simulink library "inp"  (R2021b)
settings: Solver=VariableStepAuto  StartTime=0.0  StopTime=10.0  RelTol=1e-3
undefined symbols (not defined in the file): C_TASK_5MS_S, FALSE, KINP_AcoreReadyToSlp_flg_ovrdflg, KINP_AcoreReadyToSlp_flg_ovrdval, KINP_AllowMovThd_OTA_enum_ovrdflg, KINP_AllowMovThd_OTA_enum_ovrdval, KINP_APSAngleTarget_Deg_ovrdflg, KINP_APSAngleTarget_Deg_ovrdval, KINP_APSDecReq_mps2_ovrdflg, KINP_APSDecReq_mps2_ovrdval, KINP_APSDecReqA_flg_ovrdflg, KINP_APSDecReqA_flg_ovrdval, KINP_APSDFLL_cm_ovrdflg, KINP_APSDFLL_cm_ovrdval, KINP_APSDFLR_cm_ovrdflg, KINP_APSDFLR_cm_ovrdval, KINP_APSDRLL_cm_ovrdflg, KINP_APSDRLL_cm_ovrdval, KINP_APSDRLR_cm_ovrdflg, KINP_APSDRLR_cm_ovrdval, KINP_APSExitCondition_enum_ovrdflg, KINP_APSExitCondition_enum_ovrdval, KINP_APSHWVer_enum_ovrdflg, KINP_APSHWVer_enum_ovrdval, KINP_APSProgressPCT_pct_ovrdflg, KINP_APSProgressPCT_pct_ovrdval, KINP_APSReq_enum_ovrdflg, KINP_APSReq_enum_ovrdval, KINP_APSRQDisplay_enum_ovrdflg, KINP_APSRQDisplay_enum_ovrdval, KINP_APSRqEPASCtrl_flg_ovrdflg, KINP_APSRqEPASCtrl_flg_ovrdval, KINP_APSShiftPosnReq_enum_ovrdval, KINP_APSShiftPosnReq_enum_ovrflg, KINP_APSSpeedCMD_kph_ovrdval, KINP_APSSpeedCMD_kph_ovrflg, KINP_APSStaSystem_enum_ovrdflg, KINP_APSStaSystem_enum_ovrdval, KINP_APSSWVer_enum_ovrdflg, KINP_APSSWVer_enum_ovrdval, KINP_APSVMCReqA_flg_ovrdval, KINP_APSVMCReqA_flg_ovrflg, KINP_APSVRqEPASCtrl_flg_ovrdflg, KINP_APSVRqEPASCtrl_flg_ovrdval, KINP_AuxBattVolmV_mV_ovrdflg, KINP_AuxBattVolmV_mV_ovrdval, KINP_CAASSta_enum_ovrdflg, KINP_CAASSta_enum_ovrdval, KINP_CAASVMCReqA_flg_ovrdval, KINP_CAASVMCReqA_flg_ovrflg, KINP_Chime_enum_ovrdflg, KINP_Chime_enum_ovrdval, KINP_ClearDTCcmd_flg_ovrdflg, KINP_ClearDTCcmd_flg_ovrdval, KINP_EvccAplusPwrUpReq_flg_ovrdflg, KINP_EvccAplusPwrUpReq_flg_ovrdval, KINP_LFID_raw_ovrdval, KINP_LFID_raw_ovrflg, KINP_LRID_raw_ovrdval, KINP_MemOffsetAccX_raw16_ovrdflg ... (+118)
libraries: FVT_lib x595, hcu_lib x1
(part 4 of 27)

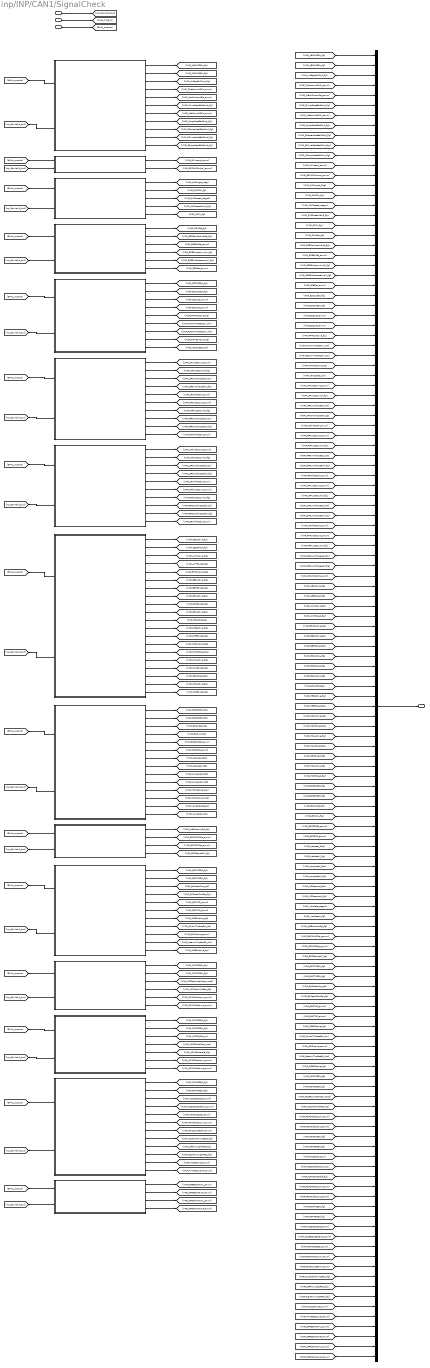
== system inp/INP/CAN1/SignalCheck ==
  inp_CanValid_bus : Inport
  TASK_TIME_S : Inport  Port=2
  BHAL_outputs : Inport  Port=3
  ABM1 : Subsystem
  EPAS1 : Subsystem
  EPAS2 : Subsystem
  EPB1 : Subsystem
  ESC1 : Subsystem
  ESC2 : Subsystem
  ESC3 : Subsystem
  ESC4 : Subsystem
  ESC5 : Subsystem
  ESC6 : Subsystem
  ESC7 : Subsystem
  FCM2 : Subsystem
  FCM3 : Subsystem
  FCM4 : Subsystem
  SRR1 : Subsystem
  bus_creator : BusCreator  Inputs=131
  inp_Hal_bus : Outport
  wires:
  inp_CanValid_bus/1 -> [inp_CanValid_bus]
  TASK_TIME_S/1 -> [TASK_TIME_S]
  BHAL_outputs/1 -> [BHAL_outputs]
  [BHAL_outputs] -> ABM1/1(BHAL_outputs)
  [inp_CanValid_bus] -> ABM1/2(inp_CanValid_bus)
  ABM1/1(VINP_ABM1CSErr_flg) -> [VINP_ABM1CSErr_flg]
  ABM1/2(VINP_ABM1RCErr_flg) -> [VINP_ABM1RCErr_flg]
  ABM1/3(VINP_AirBagFailCmd_flg) -> [VINP_AirBagFailCmd_flg]
  ABM1/4(VINP_ChecksumABM1_enum) -> [VINP_ChecksumABM1_enum]
  ABM1/5(VINP_CrashOutputSts_enum) -> [VINP_CrashOutputSts_enum]
  ABM1/6(VINP_DriverSeatBeltCmd_flg) -> [VINP_DriverSeatBeltCmd_flg]
  ABM1/7(VINP_LifeCountABM1_enum) -> [VINP_LifeCountABM1_enum]
  ABM1/8(VINP_PsngrSeatBeltCmd_flg) -> [VINP_PsngrSeatBeltCmd_flg]
  ABM1/9(VINP_RCenterSeatBeltCmd_flg) -> [VINP_RCenterSeatBeltCmd_flg]
  ABM1/10(VINP_RDriverSeatBeltCmd_flg) -> [VINP_RDriverSeatBeltCmd_flg]
  ABM1/11(VINP_RPsngrSeatBeltCmd_flg) -> [VINP_RPsngrSeatBeltCmd_flg]
  [BHAL_outputs] -> EPAS1/1(BHAL_outputs)
  [inp_CanValid_bus] -> EPAS1/2(inp_CanValid_bus)
  EPAS1/1(VINP_DriIntend_enum) -> [VINP_DriIntend_enum]
  EPAS1/2(VINP_EPSAOIControl_enum) -> [VINP_EPSAOIControl_enum]
  [BHAL_outputs] -> EPAS2/1(BHAL_outputs)
  [inp_CanValid_bus] -> EPAS2/2(inp_CanValid_bus)
  EPAS2/1(VINP_SASAngle_Deg) -> [VINP_SASAngle_Deg]
  EPAS2/2(VINP_SASCAL_flg) -> [VINP_SASCAL_flg]
  EPAS2/3(VINP_SASSpeed_degps) -> [VINP_SASSpeed_degps]
  EPAS2/4(VINP_SASSpeedValid_flg) -> [VINP_SASSpeedValid_flg]
  EPAS2/5(VINP_SASV_flg) -> [VINP_SASV_flg]
  [BHAL_outputs] -> EPB1/1(BHAL_outputs)
  [inp_CanValid_bus] -> EPB1/2(inp_CanValid_bus)
  EPB1/1(VINP_DOASta_flg) -> [VINP_DOASta_flg]
  EPB1/2(VINP_EPBCarWashMode_flg) -> [VINP_EPBCarWashMode_flg]
  EPB1/3(VINP_EPBErrSta_enum) -> [VINP_EPBErrSta_enum]
  EPB1/4(VINP_EPBExtApplyAvail_flg) -> [VINP_EPBExtApplyAvail_flg]
  EPB1/5(VINP_EPBExtReleaseAvail_flg) -> [VINP_EPBExtReleaseAvail_flg]
  EPB1/6(VINP_EPBSta_enum) -> [VINP_EPBSta_enum]
  [BHAL_outputs] -> ESC1/1(BHAL_outputs)
  [inp_CanValid_bus] -> ESC1/2(inp_CanValid_bus)
  ESC1/1(VINP_ESC1CSErr_flg) -> [VINP_ESC1CSErr_flg]
  ESC1/2(VINP_ESC1RCErr_flg) -> [VINP_ESC1RCErr_flg]
  ESC1/3(VINP_ESC1CS_enum) -> [VINP_ESC1CS_enum]
  ESC1/4(VINP_ESC1RC_enum) -> [VINP_ESC1RC_enum]
  ESC1/5(VINP_FrPTCSActive_flg) -> [VINP_FrPTCSActive_flg]
  ESC1/6(VINP_FrntAxlTrqReqDrv_Nm) -> [VINP_FrntAxlTrqReqDrv_Nm]
  ESC1/7(VINP_RearAxlTrqReqDrv_Nm) -> [VINP_RearAxlTrqReqDrv_Nm]
  ESC1/8(VINP_RrPTCSActive_flg) -> [VINP_RrPTCSActive_flg]
  ESC1/9(VINP_VehSpeed_kph) -> [VINP_VehSpeed_kph]
  [BHAL_outputs] -> ESC2/1(BHAL_outputs)
  [inp_CanValid_bus] -> ESC2/2(inp_CanValid_bus)
  ESC2/1(VINP_LFPulseCount_enum) -> [VINP_LFPulseCount_enum]
  ESC2/2(VINP_LFPulseCountV_flg) -> [VINP_LFPulseCountV_flg]
  ESC2/3(VINP_LFRawWhlSpeed_kph) -> [VINP_LFRawWhlSpeed_kph]
  ESC2/4(VINP_LFRawWhlSpeedV_flg) -> [VINP_LFRawWhlSpeedV_flg]
  ESC2/5(VINP_LFWhlRotDir_enum) -> [VINP_LFWhlRotDir_enum]
  ESC2/6(VINP_RFPulseCount_enum) -> [VINP_RFPulseCount_enum]
  ESC2/7(VINP_RFPulseCountV_flg) -> [VINP_RFPulseCountV_flg]
  ESC2/8(VINP_RFRawWhlSpeed_kph) -> [VINP_RFRawWhlSpeed_kph]
  ESC2/9(VINP_RFRawWhlSpeedV_flg) -> [VINP_RFRawWhlSpeedV_flg]
  ESC2/10(VINP_RFWhlRotDir_enum) -> [VINP_RFWhlRotDir_enum]
  [BHAL_outputs] -> ESC3/1(BHAL_outputs)
  [inp_CanValid_bus] -> ESC3/2(inp_CanValid_bus)
  ESC3/1(VINP_LRPulseCount_enum) -> [VINP_LRPulseCount_enum]
  ESC3/2(VINP_LRPulseCountV_flg) -> [VINP_LRPulseCountV_flg]
  ESC3/3(VINP_LRRawWhlSpeed_kph) -> [VINP_LRRawWhlSpeed_kph]
  ESC3/4(VINP_LRRawWhlSpeedV_flg) -> [VINP_LRRawWhlSpeedV_flg]
  ESC3/5(VINP_LRWhlRotDir_enum) -> [VINP_LRWhlRotDir_enum]
  ESC3/6(VINP_RRPulseCount_enum) -> [VINP_RRPulseCount_enum]
  ESC3/7(VINP_RRPulseCountV_flg) -> [VINP_RRPulseCountV_flg]
  ESC3/8(VINP_RRRawWhlSpeed_kph) -> [VINP_RRRawWhlSpeed_kph]
  ESC3/9(VINP_RRRawWhlSpeedV_flg) -> [VINP_RRRawWhlSpeedV_flg]
  ESC3/10(VINP_RRWhlRotDir_enum) -> [VINP_RRWhlRotDir_enum]
  [BHAL_outputs] -> ESC4/1(BHAL_outputs)
  [inp_CanValid_bus] -> ESC4/2(inp_CanValid_bus)
  ESC4/1(VINP_ABSActive_flg) -> [VINP_ABSActive_flg]
  ESC4/2(VINP_ABSFailed_flg) -> [VINP_ABSFailed_flg]
  ESC4/3(VINP_AVHActive_flg) -> [VINP_AVHActive_flg]
  ESC4/4(VINP_AVHFailed_flg) -> [VINP_AVHFailed_flg]
  ESC4/5(VINP_BTCSActive_flg) -> [VINP_BTCSActive_flg]
  ESC4/6(VINP_EBDActive_flg) -> [VINP_EBDActive_flg]
  ESC4/7(VINP_EBDFailed_flg) -> [VINP_EBDFailed_flg]
  ESC4/8(VINP_ESCActive_flg) -> [VINP_ESCActive_flg]
  ESC4/9(VINP_ESCFailed_flg) -> [VINP_ESCFailed_flg]
  ESC4/10(VINP_ESSActive_flg) -> [VINP_ESSActive_flg]
  ESC4/11(VINP_GRADE_Deg) -> [VINP_GRADE_Deg]
  ESC4/12(VINP_HBBActive_flg) -> [VINP_HBBActive_flg]
  ESC4/13(VINP_HBBFailed_flg) -> [VINP_HBBFailed_flg]
  ESC4/14(VINP_HDDActive_flg) -> [VINP_HDDActive_flg]
  ESC4/15(VINP_HDDFailed_flg) -> [VINP_HDDFailed_flg]
  ESC4/16(VINP_HSAActive_flg) -> [VINP_HSAActive_flg]
  ESC4/17(VINP_HSAFailed_flg) -> [VINP_HSAFailed_flg]
  ESC4/18(VINP_PBAFailed_flg) -> [VINP_PBAFailed_flg]
  ESC4/19(VINP_TCSActive_flg) -> [VINP_TCSActive_flg]
  ESC4/20(VINP_TCSFailed_flg) -> [VINP_TCSFailed_flg]
  [BHAL_outputs] -> ESC5/1(BHAL_outputs)
  [inp_CanValid_bus] -> ESC5/2(inp_CanValid_bus)
  ESC5/1(VINP_ESC5CSErr_flg) -> [VINP_ESC5CSErr_flg]
  ESC5/2(VINP_ESC5RCErr_flg) -> [VINP_ESC5RCErr_flg]
  ESC5/3(VINP_BrkSwSta_flg) -> [VINP_BrkSwSta_flg]
  ESC5/4(VINP_BrkSwV_flg) -> [VINP_BrkSwV_flg]
  ESC5/5(VINP_ESC5CRC8_enum) -> [VINP_ESC5CRC8_enum]
  ESC5/6(VINP_ESC5RC_enum) -> [VINP_ESC5RC_enum]
  ESC5/7(VINP_LatAccel_Gps) -> [VINP_LatAccel_Gps]
  ESC5/8(VINP_LatAccelV_flg) -> [VINP_LatAccelV_flg]
  ESC5/9(VINP_LongAccel_Gps) -> [VINP_LongAccel_Gps]
  ESC5/10(VINP_LongAccelV_flg) -> [VINP_LongAccelV_flg]
  ESC5/11(VINP_MCPressure_bar) -> [VINP_MCPressure_bar]
  ESC5/12(VINP_MCPressureV_flg) -> [VINP_MCPressureV_flg]
  ESC5/13(VINP_YawRate_degps) -> [VINP_YawRate_degps]
  ESC5/14(VINP_YawRateV_flg) -> [VINP_YawRateV_flg]
  [BHAL_outputs] -> ESC6/1(BHAL_outputs)
  [inp_CanValid_bus] -> ESC6/2(inp_CanValid_bus)
  ESC6/1(VINP_ActBrkLampSta_flg) -> [VINP_ActBrkLampSta_flg]
  ESC6/2(VINP_ESCADASSta_enum) -> [VINP_ESCADASSta_enum]
  ESC6/3(VINP_ESCAPSSta_enum) -> [VINP_ESCAPSSta_enum]
  ESC6/4(VINP_ESCStandstill_flg) -> [VINP_ESCStandstill_flg]
  [BHAL_outputs] -> ESC7/1(BHAL_outputs)
  [inp_CanValid_bus] -> ESC7/2(inp_CanValid_bus)
  ESC7/1(VINP_ESC7CSErr_flg) -> [VINP_ESC7CSErr_flg]
  ESC7/2(VINP_ESC7RCErr_flg) -> [VINP_ESC7RCErr_flg]
  ESC7/3(VINP_BrkPedalPos_pct) -> [VINP_BrkPedalPos_pct]
  ESC7/4(VINP_BrkPedalPosSta_flg) -> [VINP_BrkPedalPosSta_flg]
  ESC7/5(VINP_ESC7CS_enum) -> [VINP_ESC7CS_enum]
  ESC7/6(VINP_ESC7RC_enum) -> [VINP_ESC7RC_enum]
  ESC7/7(VINP_FrRBCActive_flg) -> [VINP_FrRBCActive_flg]
  ESC7/8(VINP_FrntAxlTrqReqBrk_Nm) -> [VINP_FrntAxlTrqReqBrk_Nm]
  ESC7/9(VINP_RDCActive_enum) -> [VINP_RDCActive_enum]
  ESC7/10(VINP_RearAxlTrqReqBrk_Nm) -> [VINP_RearAxlTrqReqBrk_Nm]
  ESC7/11(VINP_RrRBCActive_flg) -> [VINP_RrRBCActive_flg]
  [BHAL_outputs] -> FCM2/1(BHAL_outputs)
  [inp_CanValid_bus] -> FCM2/2(inp_CanValid_bus)
  FCM2/1(VINP_FCM2CSErr_flg) -> [VINP_FCM2CSErr_flg]
  FCM2/2(VINP_FCM2RCErr_flg) -> [VINP_FCM2RCErr_flg]
  FCM2/3(VINP_ACCRequiredAccel_mps2) -> [VINP_ACCRequiredAccel_mps2]
  FCM2/4(VINP_ACCVehHoldReq_flg) -> [VINP_ACCVehHoldReq_flg]
  FCM2/5(VINP_FCM2Checksum_enum) -> [VINP_FCM2Checksum_enum]
  FCM2/6(VINP_FCM2LifeCount_enum) -> [VINP_FCM2LifeCount_enum]
  [BHAL_outputs] -> FCM3/1(BHAL_outputs)
  [inp_CanValid_bus] -> FCM3/2(inp_CanValid_bus)
  FCM3/1(VINP_FCM3CSErr_flg) -> [VINP_FCM3CSErr_flg]
  FCM3/2(VINP_FCM3RCErr_flg) -> [VINP_FCM3RCErr_flg]
  FCM3/3(VINP_ACCObjDist_m) -> [VINP_ACCObjDist_m]
  FCM3/4(VINP_ACCObjRelSpd_mps) -> [VINP_ACCObjRelSpd_mps]
  FCM3/5(VINP_ADASForceIdle_flg) -> [VINP_ADASForceIdle_flg]
  FCM3/6(VINP_FCM3Checksum_enum) -> [VINP_FCM3Checksum_enum]
  FCM3/7(VINP_FCM3LifeCount_enum) -> [VINP_FCM3LifeCount_enum]
  [BHAL_outputs] -> FCM4/1(BHAL_outputs)
  [inp_CanValid_bus] -> FCM4/2(inp_CanValid_bus)
  FCM4/1(VINP_FCM4CSErr_flg) -> [VINP_FCM4CSErr_flg]
  FCM4/2(VINP_FCM4RCErr_flg) -> [VINP_FCM4RCErr_flg]
  FCM4/3(VINP_ACCSetSpeed_enum) -> [VINP_ACCSetSpeed_enum]
  FCM4/4(VINP_ACCSetSpeedDisp_enum) -> [VINP_ACCSetSpeedDisp_enum]
  FCM4/5(VINP_ADASACCSta_enum) -> [VINP_ADASACCSta_enum]
  FCM4/6(VINP_FCM4Checksum_enum) -> [VINP_FCM4Checksum_enum]
  FCM4/7(VINP_ForceLowBeam_enum) -> [VINP_ForceLowBeam_enum]
  FCM4/8(VINP_HazardWarningReq_flg) -> [VINP_HazardWarningReq_flg]
  FCM4/9(VINP_LeftTurnLightReq_flg) -> [VINP_LeftTurnLightReq_flg]
  FCM4/10(VINP_RightTurnLightReq_flg) -> [VINP_RightTurnLightReq_flg]
  FCM4/11(VINP_TargetType_enum) -> [VINP_TargetType_enum]
  FCM4/12(VINP_TimeGapLevel_enum) -> [VINP_TimeGapLevel_enum]
  [BHAL_outputs] -> SRR1/1(BHAL_outputs)
  [inp_CanValid_bus] -> SRR1/2(inp_CanValid_bus)
  SRR1/1(VINP_SRRBSDWarnL_enum) -> [VINP_SRRBSDWarnL_enum]
  SRR1/2(VINP_SRRBSDWarnR_enum) -> [VINP_SRRBSDWarnR_enum]
  SRR1/3(VINP_SRRODAWarnL_enum) -> [VINP_SRRODAWarnL_enum]
  SRR1/4(VINP_SRRODAWarnR_enum) -> [VINP_SRRODAWarnR_enum]
  bus_creator/1 -> inp_Hal_bus/1
  [VINP_ABM1CSErr_flg] -> bus_creator/1
  [VINP_ABM1RCErr_flg] -> bus_creator/2
  [VINP_AirBagFailCmd_flg] -> bus_creator/3
  [VINP_ChecksumABM1_enum] -> bus_creator/4
  [VINP_CrashOutputSts_enum] -> bus_creator/5
  [VINP_DriverSeatBeltCmd_flg] -> bus_creator/6
  [VINP_LifeCountABM1_enum] -> bus_creator/7
  [VINP_PsngrSeatBeltCmd_flg] -> bus_creator/8
  [VINP_RCenterSeatBeltCmd_flg] -> bus_creator/9
  [VINP_RDriverSeatBeltCmd_flg] -> bus_creator/10
  [VINP_RPsngrSeatBeltCmd_flg] -> bus_creator/11
  [VINP_DriIntend_enum] -> bus_creator/12
  [VINP_EPSAOIControl_enum] -> bus_creator/13
  [VINP_SASAngle_Deg] -> bus_creator/14
  [VINP_SASCAL_flg] -> bus_creator/15
  [VINP_SASSpeed_degps] -> bus_creator/16
  [VINP_SASSpeedValid_flg] -> bus_creator/17
  [VINP_SASV_flg] -> bus_creator/18
  [VINP_DOASta_flg] -> bus_creator/19
  [VINP_EPBCarWashMode_flg] -> bus_creator/20
  [VINP_EPBErrSta_enum] -> bus_creator/21
  [VINP_EPBExtApplyAvail_flg] -> bus_creator/22
  [VINP_EPBExtReleaseAvail_flg] -> bus_creator/23
  [VINP_EPBSta_enum] -> bus_creator/24
  [VINP_ESC1CSErr_flg] -> bus_creator/25
  [VINP_ESC1RCErr_flg] -> bus_creator/26
  [VINP_ESC1CS_enum] -> bus_creator/27
  [VINP_ESC1RC_enum] -> bus_creator/28
  [VINP_FrPTCSActive_flg] -> bus_creator/29
  [VINP_FrntAxlTrqReqDrv_Nm] -> bus_creator/30
  [VINP_RearAxlTrqReqDrv_Nm] -> bus_creator/31
  [VINP_RrPTCSActive_flg] -> bus_creator/32
  [VINP_VehSpeed_kph] -> bus_creator/33
  [VINP_LFPulseCount_enum] -> bus_creator/34
  [VINP_LFPulseCountV_flg] -> bus_creator/35
  [VINP_LFRawWhlSpeed_kph] -> bus_creator/36
  [VINP_LFRawWhlSpeedV_flg] -> bus_creator/37
  [VINP_LFWhlRotDir_enum] -> bus_creator/38
  [VINP_RFPulseCount_enum] -> bus_creator/39
  [VINP_RFPulseCountV_flg] -> bus_creator/40
  [VINP_RFRawWhlSpeed_kph] -> bus_creator/41
  [VINP_RFRawWhlSpeedV_flg] -> bus_creator/42
  [VINP_RFWhlRotDir_enum] -> bus_creator/43
  [VINP_LRPulseCount_enum] -> bus_creator/44
  [VINP_LRPulseCountV_flg] -> bus_creator/45
  [VINP_LRRawWhlSpeed_kph] -> bus_creator/46
  [VINP_LRRawWhlSpeedV_flg] -> bus_creator/47
  [VINP_LRWhlRotDir_enum] -> bus_creator/48
  [VINP_RRPulseCount_enum] -> bus_creator/49
  [VINP_RRPulseCountV_flg] -> bus_creator/50
  [VINP_RRRawWhlSpeed_kph] -> bus_creator/51
  [VINP_RRRawWhlSpeedV_flg] -> bus_creator/52
  [VINP_RRWhlRotDir_enum] -> bus_creator/53
  [VINP_ABSActive_flg] -> bus_creator/54
  [VINP_ABSFailed_flg] -> bus_creator/55
  [VINP_AVHActive_flg] -> bus_creator/56
  [VINP_AVHFailed_flg] -> bus_creator/57
  [VINP_BTCSActive_flg] -> bus_creator/58
  [VINP_EBDActive_flg] -> bus_creator/59
  [VINP_EBDFailed_flg] -> bus_creator/60
  [VINP_ESCActive_flg] -> bus_creator/61
  [VINP_ESCFailed_flg] -> bus_creator/62
  [VINP_ESSActive_flg] -> bus_creator/63
  [VINP_GRADE_Deg] -> bus_creator/64
  [VINP_HBBActive_flg] -> bus_creator/65
  [VINP_HBBFailed_flg] -> bus_creator/66
  [VINP_HDDActive_flg] -> bus_creator/67
  [VINP_HDDFailed_flg] -> bus_creator/68
  [VINP_HSAActive_flg] -> bus_creator/69
  [VINP_HSAFailed_flg] -> bus_creator/70
  [VINP_PBAFailed_flg] -> bus_creator/71
  [VINP_TCSActive_flg] -> bus_creator/72
  [VINP_TCSFailed_flg] -> bus_creator/73
  [VINP_ESC5CSErr_flg] -> bus_creator/74
  [VINP_ESC5RCErr_flg] -> bus_creator/75
  [VINP_BrkSwSta_flg] -> bus_creator/76
  [VINP_BrkSwV_flg] -> bus_creator/77
  [VINP_ESC5CRC8_enum] -> bus_creator/78
  [VINP_ESC5RC_enum] -> bus_creator/79
  [VINP_LatAccel_Gps] -> bus_creator/80
  [VINP_LatAccelV_flg] -> bus_creator/81
  [VINP_LongAccel_Gps] -> bus_creator/82
  [VINP_LongAccelV_flg] -> bus_creator/83
  [VINP_MCPressure_bar] -> bus_creator/84
  [VINP_MCPressureV_flg] -> bus_creator/85
  [VINP_YawRate_degps] -> bus_creator/86
  [VINP_YawRateV_flg] -> bus_creator/87
  [VINP_ActBrkLampSta_flg] -> bus_creator/88
  [VINP_ESCADASSta_enum] -> bus_creator/89
  [VINP_ESCAPSSta_enum] -> bus_creator/90
  [VINP_ESCStandstill_flg] -> bus_creator/91
  [VINP_ESC7CSErr_flg] -> bus_creator/92
  [VINP_ESC7RCErr_flg] -> bus_creator/93
  [VINP_BrkPedalPos_pct] -> bus_creator/94
  [VINP_BrkPedalPosSta_flg] -> bus_creator/95
  [VINP_ESC7CS_enum] -> bus_creator/96
  [VINP_ESC7RC_enum] -> bus_creator/97
  [VINP_FrRBCActive_flg] -> bus_creator/98
  [VINP_FrntAxlTrqReqBrk_Nm] -> bus_creator/99
  [VINP_RDCActive_enum] -> bus_creator/100
  [VINP_RearAxlTrqReqBrk_Nm] -> bus_creator/101
  [VINP_RrRBCActive_flg] -> bus_creator/102
  [VINP_FCM2CSErr_flg] -> bus_creator/103
  [VINP_FCM2RCErr_flg] -> bus_creator/104
  [VINP_ACCRequiredAccel_mps2] -> bus_creator/105
  [VINP_ACCVehHoldReq_flg] -> bus_creator/106
  [VINP_FCM2Checksum_enum] -> bus_creator/107
  [VINP_FCM2LifeCount_enum] -> bus_creator/108
  [VINP_FCM3CSErr_flg] -> bus_creator/109
  [VINP_FCM3RCErr_flg] -> bus_creator/110
  [VINP_ACCObjDist_m] -> bus_creator/111
  [VINP_ACCObjRelSpd_mps] -> bus_creator/112
  [VINP_ADASForceIdle_flg] -> bus_creator/113
  [VINP_FCM3Checksum_enum] -> bus_creator/114
  [VINP_FCM3LifeCount_enum] -> bus_creator/115
  [VINP_FCM4CSErr_flg] -> bus_creator/116
  [VINP_FCM4RCErr_flg] -> bus_creator/117
  [VINP_ACCSetSpeed_enum] -> bus_creator/118
  [VINP_ACCSetSpeedDisp_enum] -> bus_creator/119
  [VINP_ADASACCSta_enum] -> bus_creator/120
  [VINP_FCM4Checksum_enum] -> bus_creator/121
  [VINP_ForceLowBeam_enum] -> bus_creator/122
  [VINP_HazardWarningReq_flg] -> bus_creator/123
  [VINP_LeftTurnLightReq_flg] -> bus_creator/124
  [VINP_RightTurnLightReq_flg] -> bus_creator/125
  [VINP_TargetType_enum] -> bus_creator/126
  [VINP_TimeGapLevel_enum] -> bus_creator/127
  [VINP_SRRBSDWarnL_enum] -> bus_creator/128
  [VINP_SRRBSDWarnR_enum] -> bus_creator/129
  [VINP_SRRODAWarnL_enum] -> bus_creator/130
  [VINP_SRRODAWarnR_enum] -> bus_creator/131

== system inp/INP/CAN2/CommunicationCheck ==
  BHAL_outputs : Inport
  CANMsgInvalidIVI1 : FVT_lib/inp/CAN_Msg_Validity_Process_template  SystemSampleTime=-1  VariantActivationTime=update diagram  Latency=0  AutoFrameSizeCalculation=off
      link override debdec: Value=KINP_CANMsgInvalidIVI1_flg_debdec
      link override debinc: Value=KINP_CANMsgInvalidIVI1_flg_debinc
      link override deblim: Value=KINP_CANMsgInvalidIVI1_flg_deblim
      link override inverse: Value=KINP_CANMsgInvalidIVI1_flg_inverse
      link override ovrdflg: Value=KINP_CANMsgInvalidIVI1_flg_ovrdflg
      link override ovrdval: Value=KINP_CANMsgInvalidIVI1_flg_ovrdval
      link override srvcflg: Value=KINP_CANMsgInvalidIVI1_flg_srvcflg
      link override srvcval: Value=KINP_CANMsgInvalidIVI1_flg_srvcval
  CANMsgInvalidIVI2 : FVT_lib/inp/CAN_Msg_Validity_Process_template  SystemSampleTime=-1  VariantActivationTime=update diagram  Latency=0  AutoFrameSizeCalculation=off
      link override debdec: Value=KINP_CANMsgInvalidIVI2_flg_debdec
      link override debinc: Value=KINP_CANMsgInvalidIVI2_flg_debinc
      link override deblim: Value=KINP_CANMsgInvalidIVI2_flg_deblim
      link override inverse: Value=KINP_CANMsgInvalidIVI2_flg_inverse
      link override ovrdflg: Value=KINP_CANMsgInvalidIVI2_flg_ovrdflg
      link override ovrdval: Value=KINP_CANMsgInvalidIVI2_flg_ovrdval
      link override srvcflg: Value=KINP_CANMsgInvalidIVI2_flg_srvcflg
      link override srvcval: Value=KINP_CANMsgInvalidIVI2_flg_srvcval
  CANMsgInvalidIVI6 : FVT_lib/inp/CAN_Msg_Validity_Process_template  SystemSampleTime=-1  VariantActivationTime=update diagram  Latency=0  AutoFrameSizeCalculation=off
      link override debdec: Value=KINP_CANMsgInvalidIVI6_flg_debdec
      link override debinc: Value=KINP_CANMsgInvalidIVI6_flg_debinc
      link override deblim: Value=KINP_CANMsgInvalidIVI6_flg_deblim
      link override inverse: Value=KINP_CANMsgInvalidIVI6_flg_inverse
      link override ovrdflg: Value=KINP_CANMsgInvalidIVI6_flg_ovrdflg
      link override ovrdval: Value=KINP_CANMsgInvalidIVI6_flg_ovrdval
      link override srvcflg: Value=KINP_CANMsgInvalidIVI6_flg_srvcflg
      link override srvcval: Value=KINP_CANMsgInvalidIVI6_flg_srvcval
  CANMsgInvalidMETER1 : FVT_lib/inp/CAN_Msg_Validity_Process_template  SystemSampleTime=-1  VariantActivationTime=update diagram  Latency=0  AutoFrameSizeCalculation=off
      link override debdec: Value=KINP_CANMsgInvalidMETER1_flg_debdec
      link override debinc: Value=KINP_CANMsgInvalidMETER1_flg_debinc
      link override deblim: Value=KINP_CANMsgInvalidMETER1_flg_deblim
      link override inverse: Value=KINP_CANMsgInvalidMETER1_flg_inverse
      link override ovrdflg: Value=KINP_CANMsgInvalidMETER1_flg_ovrdflg
      link override ovrdval: Value=KINP_CANMsgInvalidMETER1_flg_ovrdval
      link override srvcflg: Value=KINP_CANMsgInvalidMETER1_flg_srvcflg
      link override srvcval: Value=KINP_CANMsgInvalidMETER1_flg_srvcval
  bus_creator : BusCreator  Inputs=4
  bus_selector : BusSelector  OutputSignals=VHAL_CANMsgInvalidIVI1_flg,VHAL_CANMsgInvalidIVI2_flg,VHAL_CANMsgInvalidIVI6_flg,VHAL_CANMsgInvalidMETER1_flg
  not{1..4} (4 alike) : Logic  Operator=NOT  AllPortsSameDT=off  OutDataTypeStr=boolean
  inp_CanValid_bus : Outport
  wires:
  BHAL_outputs/1 -> [BHAL_outputs]
  bus_selector/1 -> CANMsgInvalidIVI1/1  "<VHAL_CANMsgInvalidIVI1_flg>"
  CANMsgInvalidIVI1/1 -> not1/1
  not1/1 -> bus_creator/1  "VINP_CANMsgValidIVI1_flg"
  bus_selector/2 -> CANMsgInvalidIVI2/1  "<VHAL_CANMsgInvalidIVI2_flg>"
  CANMsgInvalidIVI2/1 -> not2/1
  not2/1 -> bus_creator/2  "VINP_CANMsgValidIVI2_flg"
  bus_selector/3 -> CANMsgInvalidIVI6/1  "<VHAL_CANMsgInvalidIVI6_flg>"
  CANMsgInvalidIVI6/1 -> not3/1
  not3/1 -> bus_creator/3  "VINP_CANMsgValidIVI6_flg"
  bus_selector/4 -> CANMsgInvalidMETER1/1  "<VHAL_CANMsgInvalidMETER1_flg>"
  CANMsgInvalidMETER1/1 -> not4/1
  not4/1 -> bus_creator/4  "VINP_CANMsgValidMETER1_flg"
  [BHAL_outputs] -> bus_selector/1
  bus_creator/1 -> inp_CanValid_bus/1

== system inp/INP/CAN2/CreateBus ==
  inp_CanValid_bus : Inport
  inp_Hal_bus : Inport  Port=2
  UnitConverter_{1..4,7,9..13,15,17..29,31..32,36,38..41,45,50,52,56,59..61,63..65,74,76,78..79,81,83..84,86,88..91} (53 alike) : DataTypeConversion  OutDataTypeStr=boolean
  UnitConverter_{8,14,46,66..70,77,92..93,96..102} (18 alike) : DataTypeConversion  OutDataTypeStr=single
  UnitConverter_{5..6,16,30,33..35,37,42..44,48..49,51,53..55,57..58,62,71..73,75,80,82,85,87,94..95} (30 alike) : DataTypeConversion  OutDataTypeStr=uint8
  UnitConverter_47 : DataTypeConversion  OutDataTypeStr=uint32
  bus_creator : BusCreator  Inputs=102
  bus_selector : BusSelector  OutputSignals=VINP_CANMsgValidIVI1_flg,VINP_CANMsgValidIVI2_flg,VINP_CANMsgValidIVI6_flg,VINP_CANMsgValidMETER1_flg
  bus_selector_1 : BusSelector  OutputSignals=VINP_AmbLightColorSet_enum,VINP_AmbLightUserSet_enum,VINP_BrkAbnGoReadySW_flg,VINP_DRAmbLightBrightnessSet_pct,VINP_FCPFrEvtBtnACMaxReq_flg,VINP_FCPFrEvtBtnACReq_flg,VINP_FCPFrEvtBtnAutoReq_flg,VINP_FCPFrEvtBtnSyncReq_flg,VINP_FCPMidEvtBtnAutoReq_flg,VINP_IPAmbLightBrightnessSet_pct,VINP_IVILockSoundSWSta_flg,VINP_IVIOTAUpdSta_enum,VINP_LINKtoDrive_flg,VINP_OTACancelDLReq_flg,VINP_OTACompNTFYPres_flg,VINP_OTADLReq_flg,VINP_OTASuspendDLReq_flg,VINP_OTAUpdStartReq_flg,VINP_OpenDrOpenWdoSW_flg,VINP_PWCLOSEIMD_flg,VINP_PWCONTINUEUSE_flg,VINP_SchedOTAwake_flg,VINP_SmartEcoModeSW_flg,VINP_UpdCountdownCancel_flg,VINP_UpdCountdownSkip_flg,VINP_VehACModReq_enum,VINP_AVMErrSTA_flg,VINP_AVMOFFRecButt_flg,VINP_AVMParkingmode_enum,VINP_AVMparkingcancel_enum,VINP_AVMparkingexcute_enum,VINP_ApproachUnlockSW_flg,VINP_CAASSw_enum,VINP_CDLLockButt_flg,VINP_CDLUnlockButt_flg,VINP_DSEATantiset_flg,VINP_DSEATentryfunset_flg,VINP_DSEATventreq_enum,VINP_ESCSWCmd_enum,VINP_FSOffSw_enum,VINP_FollowMeSW_flg,VINP_GPSLAT_s,VINP_GPSLONG_enum,VINP_HeadLampSW_enum,VINP_HoodLatchSW_enum,VINP_IVICreepSWReq_flg,VINP_IVIISAOffsetSpd_enum,VINP_IVINightModeSta_flg,VINP_IVIPTGModeSW_enum,VINP_IVIPTGOpenHeight_enum,VINP_IVIPTGStaSW_enum,VINP_IVIPTGUSStaSW_flg,VINP_IVIPWModeReq_enum,VINP_IVIPwrLockSW_enum,VINP_IVIPwroffreq_flg,VINP_IVIRRDefReq_flg,VINP_IVIReqV2L_flg,VINP_IVIScreen_enum,VINP_IVIStatus_flg,VINP_IVITriggerreq_flg,VINP_IVIWIMAINSW_flg,VINP_LDrvControlCommand_pct,VINP_LPasControlCommand_pct,VINP_LRLDControlCommand_pct,VINP_LRRDControlCommand_pct,VINP_MFRDNBrightReq_pct,VINP_OFFACMODE_enum,VINP_PSEATventreq_enum,VINP_PerdV2L_enum,VINP_RFogLampSW_flg,VINP_RollModeSWCmd_enum,VINP_RoomLampMode_flg,VINP_SOCV2LLimit_pct,VINP_SchedChgbutt_flg,VINP_SchedChgwake_flg,VINP_SenstivityPosition_enum,VINP_SetUnlockSingle_flg,VINP_TCSSWCmd_enum,VINP_TPMSCaliButt_flg,VINP_TPMSResButt_flg,VINP_TurnSwTimeSet_enum,VINP_WalkawayLockSW_flg,VINP_sigAirIntenZon1Req_enum,VINP_sigDfrstReq_flg,VINP_sigFaceReq_flg,VINP_sigFootReq_flg,VINP_sigRecircReq_flg,VINP_sigSetTempZon1Req_C,VINP_sigSetTempZon2Req_C,VINP_IVILocatedSTA_enum,VINP_IVITimeCheck_enum,VINP_IVITimeDay_DAY,VINP_IVITimeHour_hr,VINP_IVITimeMinute_min,VINP_IVITimeMonth_MONTH,VINP_IVITimeSecond_s,VINP_IVITimeYear_YEAR,VINP_METERKPHCalcu_kph
  BINP_outputs : Outport
  wires:
  inp_CanValid_bus/1 -> [inp_CanValid_bus]
  inp_Hal_bus/1 -> [inp_Hal_bus]
  bus_selector/1 -> UnitConverter_1/1  "<VINP_CANMsgValidIVI1_flg>"
  UnitConverter_1/1 -> bus_creator/1  "VINP_CANMsgValidIVI1_flg"
  bus_selector/2 -> UnitConverter_2/1  "<VINP_CANMsgValidIVI2_flg>"
  UnitConverter_2/1 -> bus_creator/2  "VINP_CANMsgValidIVI2_flg"
  bus_selector/3 -> UnitConverter_3/1  "<VINP_CANMsgValidIVI6_flg>"
  UnitConverter_3/1 -> bus_creator/3  "VINP_CANMsgValidIVI6_flg"
  bus_selector/4 -> UnitConverter_4/1  "<VINP_CANMsgValidMETER1_flg>"
  UnitConverter_4/1 -> bus_creator/4  "VINP_CANMsgValidMETER1_flg"
  bus_selector_1/1 -> UnitConverter_5/1  "<VINP_AmbLightColorSet_enum>"
  UnitConverter_5/1 -> bus_creator/5  "VINP_AmbLightColorSet_enum"
  bus_selector_1/2 -> UnitConverter_6/1  "<VINP_AmbLightUserSet_enum>"
  UnitConverter_6/1 -> bus_creator/6  "VINP_AmbLightUserSet_enum"
  bus_selector_1/3 -> UnitConverter_7/1  "<VINP_BrkAbnGoReadySW_flg>"
  UnitConverter_7/1 -> bus_creator/7  "VINP_BrkAbnGoReadySW_flg"
  bus_selector_1/4 -> UnitConverter_8/1  "<VINP_DRAmbLightBrightnessSet_pct>"
  UnitConverter_8/1 -> bus_creator/8  "VINP_DRAmbLightBrightnessSet_pct"
  bus_selector_1/5 -> UnitConverter_9/1  "<VINP_FCPFrEvtBtnACMaxReq_flg>"
  UnitConverter_9/1 -> bus_creator/9  "VINP_FCPFrEvtBtnACMaxReq_flg"
  bus_selector_1/6 -> UnitConverter_10/1  "<VINP_FCPFrEvtBtnACReq_flg>"
  UnitConverter_10/1 -> bus_creator/10  "VINP_FCPFrEvtBtnACReq_flg"
  bus_selector_1/7 -> UnitConverter_11/1  "<VINP_FCPFrEvtBtnAutoReq_flg>"
  UnitConverter_11/1 -> bus_creator/11  "VINP_FCPFrEvtBtnAutoReq_flg"
  bus_selector_1/8 -> UnitConverter_12/1  "<VINP_FCPFrEvtBtnSyncReq_flg>"
  UnitConverter_12/1 -> bus_creator/12  "VINP_FCPFrEvtBtnSyncReq_flg"
  bus_selector_1/9 -> UnitConverter_13/1  "<VINP_FCPMidEvtBtnAutoReq_flg>"
  UnitConverter_13/1 -> bus_creator/13  "VINP_FCPMidEvtBtnAutoReq_flg"
  bus_selector_1/10 -> UnitConverter_14/1  "<VINP_IPAmbLightBrightnessSet_pct>"
  UnitConverter_14/1 -> bus_creator/14  "VINP_IPAmbLightBrightnessSet_pct"
  bus_selector_1/11 -> UnitConverter_15/1  "<VINP_IVILockSoundSWSta_flg>"
  UnitConverter_15/1 -> bus_creator/15  "VINP_IVILockSoundSWSta_flg"
  bus_selector_1/12 -> UnitConverter_16/1  "<VINP_IVIOTAUpdSta_enum>"
  UnitConverter_16/1 -> bus_creator/16  "VINP_IVIOTAUpdSta_enum"
  bus_selector_1/13 -> UnitConverter_17/1  "<VINP_LINKtoDrive_flg>"
  UnitConverter_17/1 -> bus_creator/17  "VINP_LINKtoDrive_flg"
  bus_selector_1/14 -> UnitConverter_18/1  "<VINP_OTACancelDLReq_flg>"
  UnitConverter_18/1 -> bus_creator/18  "VINP_OTACancelDLReq_flg"
  bus_selector_1/15 -> UnitConverter_19/1  "<VINP_OTACompNTFYPres_flg>"
  UnitConverter_19/1 -> bus_creator/19  "VINP_OTACompNTFYPres_flg"
  bus_selector_1/16 -> UnitConverter_20/1  "<VINP_OTADLReq_flg>"
  UnitConverter_20/1 -> bus_creator/20  "VINP_OTADLReq_flg"
  bus_selector_1/17 -> UnitConverter_21/1  "<VINP_OTASuspendDLReq_flg>"
  UnitConverter_21/1 -> bus_creator/21  "VINP_OTASuspendDLReq_flg"
  bus_selector_1/18 -> UnitConverter_22/1  "<VINP_OTAUpdStartReq_flg>"
  UnitConverter_22/1 -> bus_creator/22  "VINP_OTAUpdStartReq_flg"
  bus_selector_1/19 -> UnitConverter_23/1  "<VINP_OpenDrOpenWdoSW_flg>"
  UnitConverter_23/1 -> bus_creator/23  "VINP_OpenDrOpenWdoSW_flg"
  bus_selector_1/20 -> UnitConverter_24/1  "<VINP_PWCLOSEIMD_flg>"
  UnitConverter_24/1 -> bus_creator/24  "VINP_PWCLOSEIMD_flg"
  bus_selector_1/21 -> UnitConverter_25/1  "<VINP_PWCONTINUEUSE_flg>"
  UnitConverter_25/1 -> bus_creator/25  "VINP_PWCONTINUEUSE_flg"
  bus_selector_1/22 -> UnitConverter_26/1  "<VINP_SchedOTAwake_flg>"
  UnitConverter_26/1 -> bus_creator/26  "VINP_SchedOTAwake_flg"
  bus_selector_1/23 -> UnitConverter_27/1  "<VINP_SmartEcoModeSW_flg>"
  UnitConverter_27/1 -> bus_creator/27  "VINP_SmartEcoModeSW_flg"
  bus_selector_1/24 -> UnitConverter_28/1  "<VINP_UpdCountdownCancel_flg>"
  UnitConverter_28/1 -> bus_creator/28  "VINP_UpdCountdownCancel_flg"
  bus_selector_1/25 -> UnitConverter_29/1  "<VINP_UpdCountdownSkip_flg>"
  UnitConverter_29/1 -> bus_creator/29  "VINP_UpdCountdownSkip_flg"
  bus_selector_1/26 -> UnitConverter_30/1  "<VINP_VehACModReq_enum>"
  UnitConverter_30/1 -> bus_creator/30  "VINP_VehACModReq_enum"
  bus_selector_1/27 -> UnitConverter_31/1  "<VINP_AVMErrSTA_flg>"
  UnitConverter_31/1 -> bus_creator/31  "VINP_AVMErrSTA_flg"
  bus_selector_1/28 -> UnitConverter_32/1  "<VINP_AVMOFFRecButt_flg>"
  UnitConverter_32/1 -> bus_creator/32  "VINP_AVMOFFRecButt_flg"
  bus_selector_1/29 -> UnitConverter_33/1  "<VINP_AVMParkingmode_enum>"
  UnitConverter_33/1 -> bus_creator/33  "VINP_AVMParkingmode_enum"
  bus_selector_1/30 -> UnitConverter_34/1  "<VINP_AVMparkingcancel_enum>"
  UnitConverter_34/1 -> bus_creator/34  "VINP_AVMparkingcancel_enum"
  bus_selector_1/31 -> UnitConverter_35/1  "<VINP_AVMparkingexcute_enum>"
  UnitConverter_35/1 -> bus_creator/35  "VINP_AVMparkingexcute_enum"
  bus_selector_1/32 -> UnitConverter_36/1  "<VINP_ApproachUnlockSW_flg>"
  UnitConverter_36/1 -> bus_creator/36  "VINP_ApproachUnlockSW_flg"
  bus_selector_1/33 -> UnitConverter_37/1  "<VINP_CAASSw_enum>"
  UnitConverter_37/1 -> bus_creator/37  "VINP_CAASSw_enum"
  bus_selector_1/34 -> UnitConverter_38/1  "<VINP_CDLLockButt_flg>"
  UnitConverter_38/1 -> bus_creator/38  "VINP_CDLLockButt_flg"
  bus_selector_1/35 -> UnitConverter_39/1  "<VINP_CDLUnlockButt_flg>"
  UnitConverter_39/1 -> bus_creator/39  "VINP_CDLUnlockButt_flg"
  bus_selector_1/36 -> UnitConverter_40/1  "<VINP_DSEATantiset_flg>"
  UnitConverter_40/1 -> bus_creator/40  "VINP_DSEATantiset_flg"
  bus_selector_1/37 -> UnitConverter_41/1  "<VINP_DSEATentryfunset_flg>"
  UnitConverter_41/1 -> bus_creator/41  "VINP_DSEATentryfunset_flg"
  bus_selector_1/38 -> UnitConverter_42/1  "<VINP_DSEATventreq_enum>"
  UnitConverter_42/1 -> bus_creator/42  "VINP_DSEATventreq_enum"
  bus_selector_1/39 -> UnitConverter_43/1  "<VINP_ESCSWCmd_enum>"
  UnitConverter_43/1 -> bus_creator/43  "VINP_ESCSWCmd_enum"
  bus_selector_1/40 -> UnitConverter_44/1  "<VINP_FSOffSw_enum>"
  UnitConverter_44/1 -> bus_creator/44  "VINP_FSOffSw_enum"
  bus_selector_1/41 -> UnitConverter_45/1  "<VINP_FollowMeSW_flg>"
  UnitConverter_45/1 -> bus_creator/45  "VINP_FollowMeSW_flg"
  bus_selector_1/42 -> UnitConverter_46/1  "<VINP_GPSLAT_s>"
  UnitConverter_46/1 -> bus_creator/46  "VINP_GPSLAT_s"
  bus_selector_1/43 -> UnitConverter_47/1  "<VINP_GPSLONG_enum>"
  UnitConverter_47/1 -> bus_creator/47  "VINP_GPSLONG_enum"
  bus_selector_1/44 -> UnitConverter_48/1  "<VINP_HeadLampSW_enum>"
  UnitConverter_48/1 -> bus_creator/48  "VINP_HeadLampSW_enum"
  bus_selector_1/45 -> UnitConverter_49/1  "<VINP_HoodLatchSW_enum>"
  UnitConverter_49/1 -> bus_creator/49  "VINP_HoodLatchSW_enum"
  bus_selector_1/46 -> UnitConverter_50/1  "<VINP_IVICreepSWReq_flg>"
  UnitConverter_50/1 -> bus_creator/50  "VINP_IVICreepSWReq_flg"
  bus_selector_1/47 -> UnitConverter_51/1  "<VINP_IVIISAOffsetSpd_enum>"
  UnitConverter_51/1 -> bus_creator/51  "VINP_IVIISAOffsetSpd_enum"
  bus_selector_1/48 -> UnitConverter_52/1  "<VINP_IVINightModeSta_flg>"
  UnitConverter_52/1 -> bus_creator/52  "VINP_IVINightModeSta_flg"
  bus_selector_1/49 -> UnitConverter_53/1  "<VINP_IVIPTGModeSW_enum>"
  UnitConverter_53/1 -> bus_creator/53  "VINP_IVIPTGModeSW_enum"
  bus_selector_1/50 -> UnitConverter_54/1  "<VINP_IVIPTGOpenHeight_enum>"
  UnitConverter_54/1 -> bus_creator/54  "VINP_IVIPTGOpenHeight_enum"
  bus_selector_1/51 -> UnitConverter_55/1  "<VINP_IVIPTGStaSW_enum>"
  UnitConverter_55/1 -> bus_creator/55  "VINP_IVIPTGStaSW_enum"
  bus_selector_1/52 -> UnitConverter_56/1  "<VINP_IVIPTGUSStaSW_flg>"
  UnitConverter_56/1 -> bus_creator/56  "VINP_IVIPTGUSStaSW_flg"
  bus_selector_1/53 -> UnitConverter_57/1  "<VINP_IVIPWModeReq_enum>"
  UnitConverter_57/1 -> bus_creator/57  "VINP_IVIPWModeReq_enum"
  bus_selector_1/54 -> UnitConverter_58/1  "<VINP_IVIPwrLockSW_enum>"
  UnitConverter_58/1 -> bus_creator/58  "VINP_IVIPwrLockSW_enum"
  bus_selector_1/55 -> UnitConverter_59/1  "<VINP_IVIPwroffreq_flg>"
  UnitConverter_59/1 -> bus_creator/59  "VINP_IVIPwroffreq_flg"
  bus_selector_1/56 -> UnitConverter_60/1  "<VINP_IVIRRDefReq_flg>"
  UnitConverter_60/1 -> bus_creator/60  "VINP_IVIRRDefReq_flg"
  bus_selector_1/57 -> UnitConverter_61/1  "<VINP_IVIReqV2L_flg>"
  UnitConverter_61/1 -> bus_creator/61  "VINP_IVIReqV2L_flg"
  bus_selector_1/58 -> UnitConverter_62/1  "<VINP_IVIScreen_enum>"
  UnitConverter_62/1 -> bus_creator/62  "VINP_IVIScreen_enum"
  bus_selector_1/59 -> UnitConverter_63/1  "<VINP_IVIStatus_flg>"
  UnitConverter_63/1 -> bus_creator/63  "VINP_IVIStatus_flg"
  bus_selector_1/60 -> UnitConverter_64/1  "<VINP_IVITriggerreq_flg>"
  UnitConverter_64/1 -> bus_creator/64  "VINP_IVITriggerreq_flg"
  bus_selector_1/61 -> UnitConverter_65/1  "<VINP_IVIWIMAINSW_flg>"
  UnitConverter_65/1 -> bus_creator/65  "VINP_IVIWIMAINSW_flg"
  bus_selector_1/62 -> UnitConverter_66/1  "<VINP_LDrvControlCommand_pct>"
  UnitConverter_66/1 -> bus_creator/66  "VINP_LDrvControlCommand_pct"
  bus_selector_1/63 -> UnitConverter_67/1  "<VINP_LPasControlCommand_pct>"
  UnitConverter_67/1 -> bus_creator/67  "VINP_LPasControlCommand_pct"
  bus_selector_1/64 -> UnitConverter_68/1  "<VINP_LRLDControlCommand_pct>"
  UnitConverter_68/1 -> bus_creator/68  "VINP_LRLDControlCommand_pct"
  bus_selector_1/65 -> UnitConverter_69/1  "<VINP_LRRDControlCommand_pct>"
  UnitConverter_69/1 -> bus_creator/69  "VINP_LRRDControlCommand_pct"
  bus_selector_1/66 -> UnitConverter_70/1  "<VINP_MFRDNBrightReq_pct>"
  UnitConverter_70/1 -> bus_creator/70  "VINP_MFRDNBrightReq_pct"
  bus_selector_1/67 -> UnitConverter_71/1  "<VINP_OFFACMODE_enum>"
  UnitConverter_71/1 -> bus_creator/71  "VINP_OFFACMODE_enum"
  bus_selector_1/68 -> UnitConverter_72/1  "<VINP_PSEATventreq_enum>"
  UnitConverter_72/1 -> bus_creator/72  "VINP_PSEATventreq_enum"
  bus_selector_1/69 -> UnitConverter_73/1  "<VINP_PerdV2L_enum>"
  UnitConverter_73/1 -> bus_creator/73  "VINP_PerdV2L_enum"
  bus_selector_1/70 -> UnitConverter_74/1  "<VINP_RFogLampSW_flg>"
  UnitConverter_74/1 -> bus_creator/74  "VINP_RFogLampSW_flg"
  bus_selector_1/71 -> UnitConverter_75/1  "<VINP_RollModeSWCmd_enum>"
  UnitConverter_75/1 -> bus_creator/75  "VINP_RollModeSWCmd_enum"
  bus_selector_1/72 -> UnitConverter_76/1  "<VINP_RoomLampMode_flg>"
  UnitConverter_76/1 -> bus_creator/76  "VINP_RoomLampMode_flg"
  bus_selector_1/73 -> UnitConverter_77/1  "<VINP_SOCV2LLimit_pct>"
  UnitConverter_77/1 -> bus_creator/77  "VINP_SOCV2LLimit_pct"
  bus_selector_1/74 -> UnitConverter_78/1  "<VINP_SchedChgbutt_flg>"
  UnitConverter_78/1 -> bus_creator/78  "VINP_SchedChgbutt_flg"
  bus_selector_1/75 -> UnitConverter_79/1  "<VINP_SchedChgwake_flg>"
  UnitConverter_79/1 -> bus_creator/79  "VINP_SchedChgwake_flg"
  bus_selector_1/76 -> UnitConverter_80/1  "<VINP_SenstivityPosition_enum>"
  UnitConverter_80/1 -> bus_creator/80  "VINP_SenstivityPosition_enum"
  bus_selector_1/77 -> UnitConverter_81/1  "<VINP_SetUnlockSingle_flg>"
  UnitConverter_81/1 -> bus_creator/81  "VINP_SetUnlockSingle_flg"
  bus_selector_1/78 -> UnitConverter_82/1  "<VINP_TCSSWCmd_enum>"
  UnitConverter_82/1 -> bus_creator/82  "VINP_TCSSWCmd_enum"
  bus_selector_1/79 -> UnitConverter_83/1  "<VINP_TPMSCaliButt_flg>"
  UnitConverter_83/1 -> bus_creator/83  "VINP_TPMSCaliButt_flg"
  bus_selector_1/80 -> UnitConverter_84/1  "<VINP_TPMSResButt_flg>"
  UnitConverter_84/1 -> bus_creator/84  "VINP_TPMSResButt_flg"
  bus_selector_1/81 -> UnitConverter_85/1  "<VINP_TurnSwTimeSet_enum>"
  UnitConverter_85/1 -> bus_creator/85  "VINP_TurnSwTimeSet_enum"
  bus_selector_1/82 -> UnitConverter_86/1  "<VINP_WalkawayLockSW_flg>"
  UnitConverter_86/1 -> bus_creator/86  "VINP_WalkawayLockSW_flg"
  bus_selector_1/83 -> UnitConverter_87/1  "<VINP_sigAirIntenZon1Req_enum>"
  UnitConverter_87/1 -> bus_creator/87  "VINP_sigAirIntenZon1Req_enum"
  bus_selector_1/84 -> UnitConverter_88/1  "<VINP_sigDfrstReq_flg>"
  UnitConverter_88/1 -> bus_creator/88  "VINP_sigDfrstReq_flg"
  bus_selector_1/85 -> UnitConverter_89/1  "<VINP_sigFaceReq_flg>"
  UnitConverter_89/1 -> bus_creator/89  "VINP_sigFaceReq_flg"
  bus_selector_1/86 -> UnitConverter_90/1  "<VINP_sigFootReq_flg>"
  UnitConverter_90/1 -> bus_creator/90  "VINP_sigFootReq_flg"
  bus_selector_1/87 -> UnitConverter_91/1  "<VINP_sigRecircReq_flg>"
  UnitConverter_91/1 -> bus_creator/91  "VINP_sigRecircReq_flg"
  bus_selector_1/88 -> UnitConverter_92/1  "<VINP_sigSetTempZon1Req_C>"
  UnitConverter_92/1 -> bus_creator/92  "VINP_sigSetTempZon1Req_C"
  bus_selector_1/89 -> UnitConverter_93/1  "<VINP_sigSetTempZon2Req_C>"
  UnitConverter_93/1 -> bus_creator/93  "VINP_sigSetTempZon2Req_C"
  bus_selector_1/90 -> UnitConverter_94/1  "<VINP_IVILocatedSTA_enum>"
  UnitConverter_94/1 -> bus_creator/94  "VINP_IVILocatedSTA_enum"
  bus_selector_1/91 -> UnitConverter_95/1  "<VINP_IVITimeCheck_enum>"
  UnitConverter_95/1 -> bus_creator/95  "VINP_IVITimeCheck_enum"
  bus_selector_1/92 -> UnitConverter_96/1  "<VINP_IVITimeDay_DAY>"
  UnitConverter_96/1 -> bus_creator/96  "VINP_IVITimeDay_DAY"
  bus_selector_1/93 -> UnitConverter_97/1  "<VINP_IVITimeHour_hr>"
  UnitConverter_97/1 -> bus_creator/97  "VINP_IVITimeHour_hr"
  bus_selector_1/94 -> UnitConverter_98/1  "<VINP_IVITimeMinute_min>"
  UnitConverter_98/1 -> bus_creator/98  "VINP_IVITimeMinute_min"
  bus_selector_1/95 -> UnitConverter_99/1  "<VINP_IVITimeMonth_MONTH>"
  UnitConverter_99/1 -> bus_creator/99  "VINP_IVITimeMonth_MONTH"
  bus_selector_1/96 -> UnitConverter_100/1  "<VINP_IVITimeSecond_s>"
  UnitConverter_100/1 -> bus_creator/100  "VINP_IVITimeSecond_s"
  bus_selector_1/97 -> UnitConverter_101/1  "<VINP_IVITimeYear_YEAR>"
  UnitConverter_101/1 -> bus_creator/101  "VINP_IVITimeYear_YEAR"
  bus_selector_1/98 -> UnitConverter_102/1  "<VINP_METERKPHCalcu_kph>"
  UnitConverter_102/1 -> bus_creator/102  "VINP_METERKPHCalcu_kph"
  [inp_CanValid_bus] -> bus_selector/1
  [inp_Hal_bus] -> bus_selector_1/1
  bus_creator/1 -> BINP_outputs/1

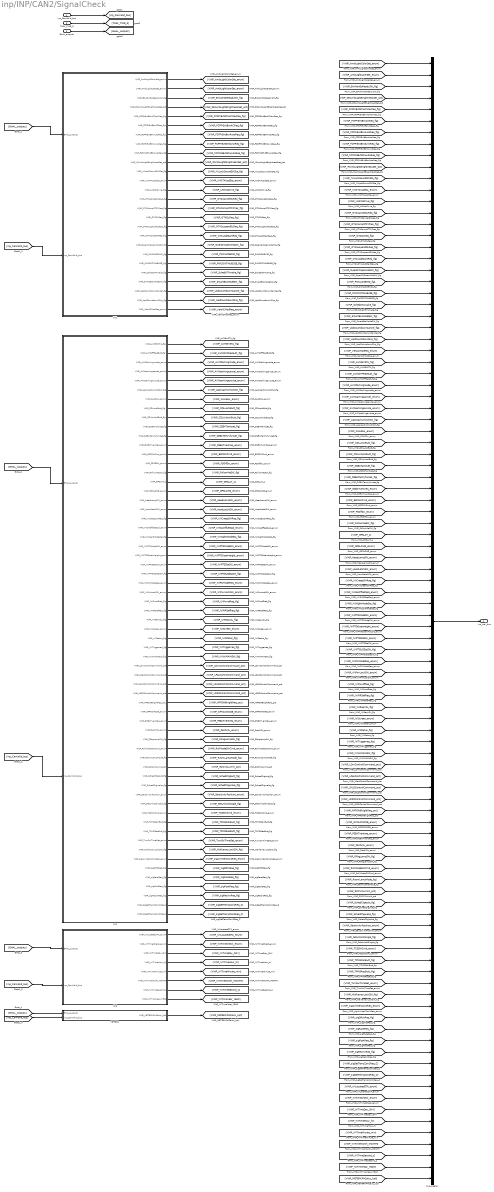
== system inp/INP/CAN2/SignalCheck ==
  inp_CanValid_bus : Inport
  TASK_TIME_S : Inport  Port=2
  BHAL_outputs : Inport  Port=3
  IVI1 : Subsystem
  IVI2 : Subsystem
  IVI6 : Subsystem
  METER1 : Subsystem
  bus_creator : BusCreator  Inputs=98
  inp_Hal_bus : Outport
  wires:
  inp_CanValid_bus/1 -> [inp_CanValid_bus]
  TASK_TIME_S/1 -> [TASK_TIME_S]
  BHAL_outputs/1 -> [BHAL_outputs]
  [BHAL_outputs] -> IVI1/1(BHAL_outputs)
  [inp_CanValid_bus] -> IVI1/2(inp_CanValid_bus)
  IVI1/1(VINP_AmbLightColorSet_enum) -> [VINP_AmbLightColorSet_enum]
  IVI1/2(VINP_AmbLightUserSet_enum) -> [VINP_AmbLightUserSet_enum]
  IVI1/3(VINP_BrkAbnGoReadySW_flg) -> [VINP_BrkAbnGoReadySW_flg]
  IVI1/4(VINP_DRAmbLightBrightnessSet_pct) -> [VINP_DRAmbLightBrightnessSet_pct]
  IVI1/5(VINP_FCPFrEvtBtnACMaxReq_flg) -> [VINP_FCPFrEvtBtnACMaxReq_flg]
  IVI1/6(VINP_FCPFrEvtBtnACReq_flg) -> [VINP_FCPFrEvtBtnACReq_flg]
  IVI1/7(VINP_FCPFrEvtBtnAutoReq_flg) -> [VINP_FCPFrEvtBtnAutoReq_flg]
  IVI1/8(VINP_FCPFrEvtBtnSyncReq_flg) -> [VINP_FCPFrEvtBtnSyncReq_flg]
  IVI1/9(VINP_FCPMidEvtBtnAutoReq_flg) -> [VINP_FCPMidEvtBtnAutoReq_flg]
  IVI1/10(VINP_IPAmbLightBrightnessSet_pct) -> [VINP_IPAmbLightBrightnessSet_pct]
  IVI1/11(VINP_IVILockSoundSWSta_flg) -> [VINP_IVILockSoundSWSta_flg]
  IVI1/12(VINP_IVIOTAUpdSta_enum) -> [VINP_IVIOTAUpdSta_enum]
  IVI1/13(VINP_LINKtoDrive_flg) -> [VINP_LINKtoDrive_flg]
  IVI1/14(VINP_OTACancelDLReq_flg) -> [VINP_OTACancelDLReq_flg]
  IVI1/15(VINP_OTACompNTFYPres_flg) -> [VINP_OTACompNTFYPres_flg]
  IVI1/16(VINP_OTADLReq_flg) -> [VINP_OTADLReq_flg]
  IVI1/17(VINP_OTASuspendDLReq_flg) -> [VINP_OTASuspendDLReq_flg]
  IVI1/18(VINP_OTAUpdStartReq_flg) -> [VINP_OTAUpdStartReq_flg]
  IVI1/19(VINP_OpenDrOpenWdoSW_flg) -> [VINP_OpenDrOpenWdoSW_flg]
  IVI1/20(VINP_PWCLOSEIMD_flg) -> [VINP_PWCLOSEIMD_flg]
  IVI1/21(VINP_PWCONTINUEUSE_flg) -> [VINP_PWCONTINUEUSE_flg]
  IVI1/22(VINP_SchedOTAwake_flg) -> [VINP_SchedOTAwake_flg]
  IVI1/23(VINP_SmartEcoModeSW_flg) -> [VINP_SmartEcoModeSW_flg]
  IVI1/24(VINP_UpdCountdownCancel_flg) -> [VINP_UpdCountdownCancel_flg]
  IVI1/25(VINP_UpdCountdownSkip_flg) -> [VINP_UpdCountdownSkip_flg]
  IVI1/26(VINP_VehACModReq_enum) -> [VINP_VehACModReq_enum]
  [BHAL_outputs] -> IVI2/1(BHAL_outputs)
  [inp_CanValid_bus] -> IVI2/2(inp_CanValid_bus)
  IVI2/1(VINP_AVMErrSTA_flg) -> [VINP_AVMErrSTA_flg]
  IVI2/2(VINP_AVMOFFRecButt_flg) -> [VINP_AVMOFFRecButt_flg]
  IVI2/3(VINP_AVMParkingmode_enum) -> [VINP_AVMParkingmode_enum]
  IVI2/4(VINP_AVMparkingcancel_enum) -> [VINP_AVMparkingcancel_enum]
  IVI2/5(VINP_AVMparkingexcute_enum) -> [VINP_AVMparkingexcute_enum]
  IVI2/6(VINP_ApproachUnlockSW_flg) -> [VINP_ApproachUnlockSW_flg]
  IVI2/7(VINP_CAASSw_enum) -> [VINP_CAASSw_enum]
  IVI2/8(VINP_CDLLockButt_flg) -> [VINP_CDLLockButt_flg]
  IVI2/9(VINP_CDLUnlockButt_flg) -> [VINP_CDLUnlockButt_flg]
  IVI2/10(VINP_DSEATantiset_flg) -> [VINP_DSEATantiset_flg]
  IVI2/11(VINP_DSEATentryfunset_flg) -> [VINP_DSEATentryfunset_flg]
  IVI2/12(VINP_DSEATventreq_enum) -> [VINP_DSEATventreq_enum]
  IVI2/13(VINP_ESCSWCmd_enum) -> [VINP_ESCSWCmd_enum]
  IVI2/14(VINP_FSOffSw_enum) -> [VINP_FSOffSw_enum]
  IVI2/15(VINP_FollowMeSW_flg) -> [VINP_FollowMeSW_flg]
  IVI2/16(VINP_GPSLAT_s) -> [VINP_GPSLAT_s]
  IVI2/17(VINP_GPSLONG_enum) -> [VINP_GPSLONG_enum]
  IVI2/18(VINP_HeadLampSW_enum) -> [VINP_HeadLampSW_enum]
  IVI2/19(VINP_HoodLatchSW_enum) -> [VINP_HoodLatchSW_enum]
  IVI2/20(VINP_IVICreepSWReq_flg) -> [VINP_IVICreepSWReq_flg]
  IVI2/21(VINP_IVIISAOffsetSpd_enum) -> [VINP_IVIISAOffsetSpd_enum]
  IVI2/22(VINP_IVINightModeSta_flg) -> [VINP_IVINightModeSta_flg]
  IVI2/23(VINP_IVIPTGModeSW_enum) -> [VINP_IVIPTGModeSW_enum]
  IVI2/24(VINP_IVIPTGOpenHeight_enum) -> [VINP_IVIPTGOpenHeight_enum]
  IVI2/25(VINP_IVIPTGStaSW_enum) -> [VINP_IVIPTGStaSW_enum]
  IVI2/26(VINP_IVIPTGUSStaSW_flg) -> [VINP_IVIPTGUSStaSW_flg]
  IVI2/27(VINP_IVIPWModeReq_enum) -> [VINP_IVIPWModeReq_enum]
  IVI2/28(VINP_IVIPwrLockSW_enum) -> [VINP_IVIPwrLockSW_enum]
  IVI2/29(VINP_IVIPwroffreq_flg) -> [VINP_IVIPwroffreq_flg]
  IVI2/30(VINP_IVIRRDefReq_flg) -> [VINP_IVIRRDefReq_flg]
  IVI2/31(VINP_IVIReqV2L_flg) -> [VINP_IVIReqV2L_flg]
  IVI2/32(VINP_IVIScreen_enum) -> [VINP_IVIScreen_enum]
  IVI2/33(VINP_IVIStatus_flg) -> [VINP_IVIStatus_flg]
  IVI2/34(VINP_IVITriggerreq_flg) -> [VINP_IVITriggerreq_flg]
  IVI2/35(VINP_IVIWIMAINSW_flg) -> [VINP_IVIWIMAINSW_flg]
  IVI2/36(VINP_LDrvControlCommand_pct) -> [VINP_LDrvControlCommand_pct]
  IVI2/37(VINP_LPasControlCommand_pct) -> [VINP_LPasControlCommand_pct]
  IVI2/38(VINP_LRLDControlCommand_pct) -> [VINP_LRLDControlCommand_pct]
  IVI2/39(VINP_LRRDControlCommand_pct) -> [VINP_LRRDControlCommand_pct]
  IVI2/40(VINP_MFRDNBrightReq_pct) -> [VINP_MFRDNBrightReq_pct]
  IVI2/41(VINP_OFFACMODE_enum) -> [VINP_OFFACMODE_enum]
  IVI2/42(VINP_PSEATventreq_enum) -> [VINP_PSEATventreq_enum]
  IVI2/43(VINP_PerdV2L_enum) -> [VINP_PerdV2L_enum]
  IVI2/44(VINP_RFogLampSW_flg) -> [VINP_RFogLampSW_flg]
  IVI2/45(VINP_RollModeSWCmd_enum) -> [VINP_RollModeSWCmd_enum]
  IVI2/46(VINP_RoomLampMode_flg) -> [VINP_RoomLampMode_flg]
  IVI2/47(VINP_SOCV2LLimit_pct) -> [VINP_SOCV2LLimit_pct]
  IVI2/48(VINP_SchedChgbutt_flg) -> [VINP_SchedChgbutt_flg]
  IVI2/49(VINP_SchedChgwake_flg) -> [VINP_SchedChgwake_flg]
  IVI2/50(VINP_SenstivityPosition_enum) -> [VINP_SenstivityPosition_enum]
  IVI2/51(VINP_SetUnlockSingle_flg) -> [VINP_SetUnlockSingle_flg]
  IVI2/52(VINP_TCSSWCmd_enum) -> [VINP_TCSSWCmd_enum]
  IVI2/53(VINP_TPMSCaliButt_flg) -> [VINP_TPMSCaliButt_flg]
  IVI2/54(VINP_TPMSResButt_flg) -> [VINP_TPMSResButt_flg]
  IVI2/55(VINP_TurnSwTimeSet_enum) -> [VINP_TurnSwTimeSet_enum]
  IVI2/56(VINP_WalkawayLockSW_flg) -> [VINP_WalkawayLockSW_flg]
  IVI2/57(VINP_sigAirIntenZon1Req_enum) -> [VINP_sigAirIntenZon1Req_enum]
  IVI2/58(VINP_sigDfrstReq_flg) -> [VINP_sigDfrstReq_flg]
  IVI2/59(VINP_sigFaceReq_flg) -> [VINP_sigFaceReq_flg]
  IVI2/60(VINP_sigFootReq_flg) -> [VINP_sigFootReq_flg]
  IVI2/61(VINP_sigRecircReq_flg) -> [VINP_sigRecircReq_flg]
  IVI2/62(VINP_sigSetTempZon1Req_C) -> [VINP_sigSetTempZon1Req_C]
  IVI2/63(VINP_sigSetTempZon2Req_C) -> [VINP_sigSetTempZon2Req_C]
  [BHAL_outputs] -> IVI6/1(BHAL_outputs)
  [inp_CanValid_bus] -> IVI6/2(inp_CanValid_bus)
  IVI6/1(VINP_IVILocatedSTA_enum) -> [VINP_IVILocatedSTA_enum]
  IVI6/2(VINP_IVITimeCheck_enum) -> [VINP_IVITimeCheck_enum]
  IVI6/3(VINP_IVITimeDay_DAY) -> [VINP_IVITimeDay_DAY]
  IVI6/4(VINP_IVITimeHour_hr) -> [VINP_IVITimeHour_hr]
  IVI6/5(VINP_IVITimeMinute_min) -> [VINP_IVITimeMinute_min]
  IVI6/6(VINP_IVITimeMonth_MONTH) -> [VINP_IVITimeMonth_MONTH]
  IVI6/7(VINP_IVITimeSecond_s) -> [VINP_IVITimeSecond_s]
  IVI6/8(VINP_IVITimeYear_YEAR) -> [VINP_IVITimeYear_YEAR]
  [BHAL_outputs] -> METER1/1(BHAL_outputs)
  [inp_CanValid_bus] -> METER1/2(inp_CanValid_bus)
  METER1/1(VINP_METERKPHCalcu_kph) -> [VINP_METERKPHCalcu_kph]
  bus_creator/1 -> inp_Hal_bus/1
  [VINP_AmbLightColorSet_enum] -> bus_creator/1
  [VINP_AmbLightUserSet_enum] -> bus_creator/2
  [VINP_BrkAbnGoReadySW_flg] -> bus_creator/3
  [VINP_DRAmbLightBrightnessSet_pct] -> bus_creator/4
  [VINP_FCPFrEvtBtnACMaxReq_flg] -> bus_creator/5
  [VINP_FCPFrEvtBtnACReq_flg] -> bus_creator/6
  [VINP_FCPFrEvtBtnAutoReq_flg] -> bus_creator/7
  [VINP_FCPFrEvtBtnSyncReq_flg] -> bus_creator/8
  [VINP_FCPMidEvtBtnAutoReq_flg] -> bus_creator/9
  [VINP_IPAmbLightBrightnessSet_pct] -> bus_creator/10
  [VINP_IVILockSoundSWSta_flg] -> bus_creator/11
  [VINP_IVIOTAUpdSta_enum] -> bus_creator/12
  [VINP_LINKtoDrive_flg] -> bus_creator/13
  [VINP_OTACancelDLReq_flg] -> bus_creator/14
  [VINP_OTACompNTFYPres_flg] -> bus_creator/15
  [VINP_OTADLReq_flg] -> bus_creator/16
  [VINP_OTASuspendDLReq_flg] -> bus_creator/17
  [VINP_OTAUpdStartReq_flg] -> bus_creator/18
  [VINP_OpenDrOpenWdoSW_flg] -> bus_creator/19
  [VINP_PWCLOSEIMD_flg] -> bus_creator/20
  [VINP_PWCONTINUEUSE_flg] -> bus_creator/21
  [VINP_SchedOTAwake_flg] -> bus_creator/22
  [VINP_SmartEcoModeSW_flg] -> bus_creator/23
  [VINP_UpdCountdownCancel_flg] -> bus_creator/24
  [VINP_UpdCountdownSkip_flg] -> bus_creator/25
  [VINP_VehACModReq_enum] -> bus_creator/26
  [VINP_AVMErrSTA_flg] -> bus_creator/27
  [VINP_AVMOFFRecButt_flg] -> bus_creator/28
  [VINP_AVMParkingmode_enum] -> bus_creator/29
  [VINP_AVMparkingcancel_enum] -> bus_creator/30
  [VINP_AVMparkingexcute_enum] -> bus_creator/31
  [VINP_ApproachUnlockSW_flg] -> bus_creator/32
  [VINP_CAASSw_enum] -> bus_creator/33
  [VINP_CDLLockButt_flg] -> bus_creator/34
  [VINP_CDLUnlockButt_flg] -> bus_creator/35
  [VINP_DSEATantiset_flg] -> bus_creator/36
  [VINP_DSEATentryfunset_flg] -> bus_creator/37
  [VINP_DSEATventreq_enum] -> bus_creator/38
  [VINP_ESCSWCmd_enum] -> bus_creator/39
  [VINP_FSOffSw_enum] -> bus_creator/40
  [VINP_FollowMeSW_flg] -> bus_creator/41
  [VINP_GPSLAT_s] -> bus_creator/42
  [VINP_GPSLONG_enum] -> bus_creator/43
  [VINP_HeadLampSW_enum] -> bus_creator/44
  [VINP_HoodLatchSW_enum] -> bus_creator/45
  [VINP_IVICreepSWReq_flg] -> bus_creator/46
  [VINP_IVIISAOffsetSpd_enum] -> bus_creator/47
  [VINP_IVINightModeSta_flg] -> bus_creator/48
  [VINP_IVIPTGModeSW_enum] -> bus_creator/49
  [VINP_IVIPTGOpenHeight_enum] -> bus_creator/50
  [VINP_IVIPTGStaSW_enum] -> bus_creator/51
  [VINP_IVIPTGUSStaSW_flg] -> bus_creator/52
  [VINP_IVIPWModeReq_enum] -> bus_creator/53
  [VINP_IVIPwrLockSW_enum] -> bus_creator/54
  [VINP_IVIPwroffreq_flg] -> bus_creator/55
  [VINP_IVIRRDefReq_flg] -> bus_creator/56
  [VINP_IVIReqV2L_flg] -> bus_creator/57
  [VINP_IVIScreen_enum] -> bus_creator/58
  [VINP_IVIStatus_flg] -> bus_creator/59
  [VINP_IVITriggerreq_flg] -> bus_creator/60
  [VINP_IVIWIMAINSW_flg] -> bus_creator/61
  [VINP_LDrvControlCommand_pct] -> bus_creator/62
  [VINP_LPasControlCommand_pct] -> bus_creator/63
  [VINP_LRLDControlCommand_pct] -> bus_creator/64
  [VINP_LRRDControlCommand_pct] -> bus_creator/65
  [VINP_MFRDNBrightReq_pct] -> bus_creator/66
  [VINP_OFFACMODE_enum] -> bus_creator/67
  [VINP_PSEATventreq_enum] -> bus_creator/68
  [VINP_PerdV2L_enum] -> bus_creator/69
  [VINP_RFogLampSW_flg] -> bus_creator/70
  [VINP_RollModeSWCmd_enum] -> bus_creator/71
  [VINP_RoomLampMode_flg] -> bus_creator/72
  [VINP_SOCV2LLimit_pct] -> bus_creator/73
  [VINP_SchedChgbutt_flg] -> bus_creator/74
  [VINP_SchedChgwake_flg] -> bus_creator/75
  [VINP_SenstivityPosition_enum] -> bus_creator/76
  [VINP_SetUnlockSingle_flg] -> bus_creator/77
  [VINP_TCSSWCmd_enum] -> bus_creator/78
  [VINP_TPMSCaliButt_flg] -> bus_creator/79
  [VINP_TPMSResButt_flg] -> bus_creator/80
  [VINP_TurnSwTimeSet_enum] -> bus_creator/81
  [VINP_WalkawayLockSW_flg] -> bus_creator/82
  [VINP_sigAirIntenZon1Req_enum] -> bus_creator/83
  [VINP_sigDfrstReq_flg] -> bus_creator/84
  [VINP_sigFaceReq_flg] -> bus_creator/85
  [VINP_sigFootReq_flg] -> bus_creator/86
  [VINP_sigRecircReq_flg] -> bus_creator/87
  [VINP_sigSetTempZon1Req_C] -> bus_creator/88
  [VINP_sigSetTempZon2Req_C] -> bus_creator/89
  [VINP_IVILocatedSTA_enum] -> bus_creator/90
  [VINP_IVITimeCheck_enum] -> bus_creator/91
  [VINP_IVITimeDay_DAY] -> bus_creator/92
  [VINP_IVITimeHour_hr] -> bus_creator/93
  [VINP_IVITimeMinute_min] -> bus_creator/94
  [VINP_IVITimeMonth_MONTH] -> bus_creator/95
  [VINP_IVITimeSecond_s] -> bus_creator/96
  [VINP_IVITimeYear_YEAR] -> bus_creator/97
  [VINP_METERKPHCalcu_kph] -> bus_creator/98
